simulink model "RCAMSimulation"  (R2018b)
settings: Solver=VariableStepAuto  StartTime=0.0  StopTime=TF  RelTol=1e-3
values from neighbouring files (symbols this model uses):
  u1max = 25*pi/180    (= 0.436332312999)    [InitializeConstants.m]
  u1min = -25*pi/180    (= -0.436332312999)    [InitializeConstants.m]
  u2max = 10*pi/180    (= 0.174532925199)    [InitializeConstants.m]
  u2min = -25*pi/180    (= -0.436332312999)    [InitializeConstants.m]
  u3max = 30*pi/180    (= 0.523598775598)    [InitializeConstants.m]
  u3min = -30*pi/180    (= -0.523598775598)    [InitializeConstants.m]
  u4max = 10*pi/180    (= 0.174532925199)    [InitializeConstants.m]
  u4min = -0.5*pi/180    (= -0.00872664625997)    [InitializeConstants.m]
  u5max = 10*pi/180    (= 0.174532925199)    [InitializeConstants.m]
  u5min = -0.5*pi/180    (= -0.00872664625997)    [InitializeConstants.m]
  x0 = [85 ... (first row only)    [InitializeConstants.m]
undefined symbols (not defined in the file or in its folder): RCAM_model
settings Model: Creator=abc  LastModifiedBy=abc

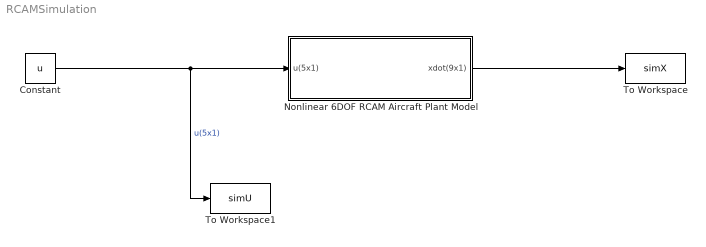
== system RCAMSimulation ==
  Constant : Constant  Value=u
  Nonlinear 6DOF RCAM Aircraft Plant Model : Subsystem
  To Workspace : ToWorkspace  VariableName=simX  SaveFormat=Timeseries  SampleTime=-1
  To Workspace1 : ToWorkspace  VariableName=simU  SaveFormat=Timeseries  SampleTime=-1
  wires:
  Constant/1 -> To Workspace1/1, Nonlinear 6DOF RCAM Aircraft Plant Model/1(u(5x1))  "u(5x1)"
  Nonlinear 6DOF RCAM Aircraft Plant Model/1(xdot(9x1)) -> To Workspace/1

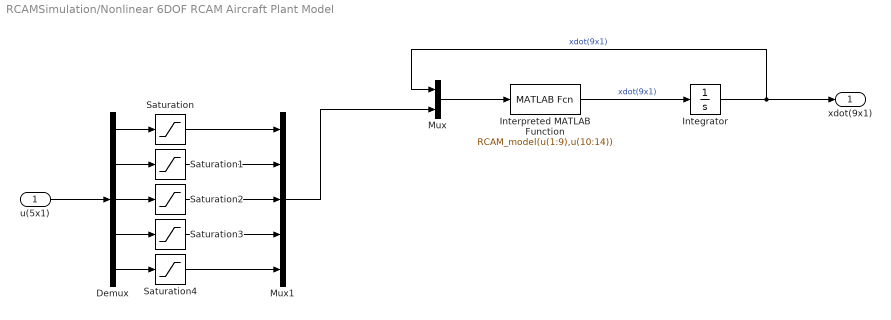
== system RCAMSimulation/Nonlinear 6DOF RCAM Aircraft Plant Model ==
  u(5x1) : Inport
  Demux : Demux  Outputs=5
  Integrator : Integrator  InitialCondition=x0
  Interpreted MATLAB Function : MATLABFcn  MATLABFcn=RCAM_model(u(1:9),u(10:14))
  Mux : Mux  Inputs=2
  Mux1 : Mux  Inputs=5
  Saturation : Saturate  UpperLimit=u1max  LowerLimit=u1min
  Saturation1 : Saturate  UpperLimit=u2max  LowerLimit=u2min
  Saturation2 : Saturate  UpperLimit=u3max  LowerLimit=u3min
  Saturation3 : Saturate  UpperLimit=u4max  LowerLimit=u4min
  Saturation4 : Saturate  UpperLimit=u5max  LowerLimit=u5min
  xdot(9x1) : Outport
  wires:
  Integrator/1 -> xdot(9x1)/1, Mux/1  "xdot(9x1)"
  Mux/1 -> Interpreted MATLAB Function/1
  Interpreted MATLAB Function/1 -> Integrator/1  "xdot(9x1)"
  u(5x1)/1 -> Demux/1
  Demux/1 -> Saturation/1
  Demux/2 -> Saturation1/1
  Demux/3 -> Saturation2/1
  Demux/4 -> Saturation3/1
  Demux/5 -> Saturation4/1
  Mux1/1 -> Mux/2
  Saturation/1 -> Mux1/1
  Saturation1/1 -> Mux1/2
  Saturation2/1 -> Mux1/3
  Saturation3/1 -> Mux1/4
  Saturation4/1 -> Mux1/5
